simulink model "ask3"  (R2016a)
settings: Solver=VariableStepAuto  StartTime=0.0  StopTime=0.2  RelTol=1e-3
values from neighbouring files (symbols this model uses):
  kd3 = kp3*Td    (= 0.002508741)    [ex1.m]
  ki3 = kp3/Ti    (= 16.0871528562)    [ex1.m]
  kp3 = 0.57    [ex1.m]
libraries: simulink x1
settings Model: Creator=JIM  LastModifiedBy=JIM

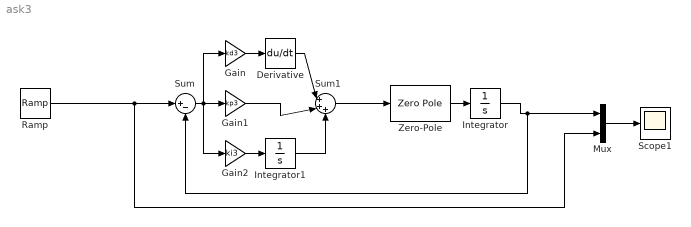
== system ask3 ==
  Derivative : Derivative
  Gain : Gain  Gain=kd3
  Gain1 : Gain  Gain=kp3
  Gain2 : Gain  Gain=ki3
  Integrator : Integrator
  Integrator1 : Integrator
  Mux : Mux  Inputs=2
  Ramp : simulink/Sources/Ramp  slope=1  start=0  X0=0
  Scope1 : Scope
  Sum : Sum  Inputs=|+-
  Sum1 : Sum  Inputs=|+++
  Zero-Pole : ZeroPole  Zeros=[0]  Poles="[0  -400.26 -3008]"  Gain=[2.717*10^9]
  wires:
  Sum/1 -> Gain/1, Gain2/1, Gain1/1
  Mux/1 -> Scope1/1
  Zero-Pole/1 -> Integrator/1
  Integrator/1 -> Sum/2, Mux/1
  Gain2/1 -> Integrator1/1
  Gain/1 -> Derivative/1
  Derivative/1 -> Sum1/1
  Gain1/1 -> Sum1/2
  Integrator1/1 -> Sum1/3
  Sum1/1 -> Zero-Pole/1
  Ramp/1 -> Mux/2, Sum/1
